simulink model "7. Ramp"  (R2017a)
settings: Solver=VariableStepAuto  StartTime=0.0  StopTime=10.0  RelTol=1e-3
libraries: simulink x1
settings Model: Creator=nardone2u  LastModifiedBy=nardone2u

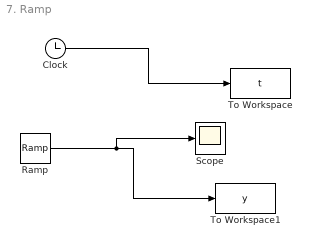
== system 7. Ramp ==
  Clock : Clock
  Ramp : simulink/Sources/Ramp  slope=0.5  start=0  X0=0
  Scope : Scope
  To Workspace : ToWorkspace  VariableName=t  SampleTime=-1
  To Workspace1 : ToWorkspace  VariableName=y  SampleTime=-1
  wires:
  Ramp/1 -> Scope/1, To Workspace1/1
  Clock/1 -> To Workspace/1
